simulink model "cocospec_2"  (R2015a)
settings: Solver=ode45  StartTime=0.0  StopTime=10.0  RelTol=1e-3
settings Model: Creator=teme  LastModifiedBy=teme

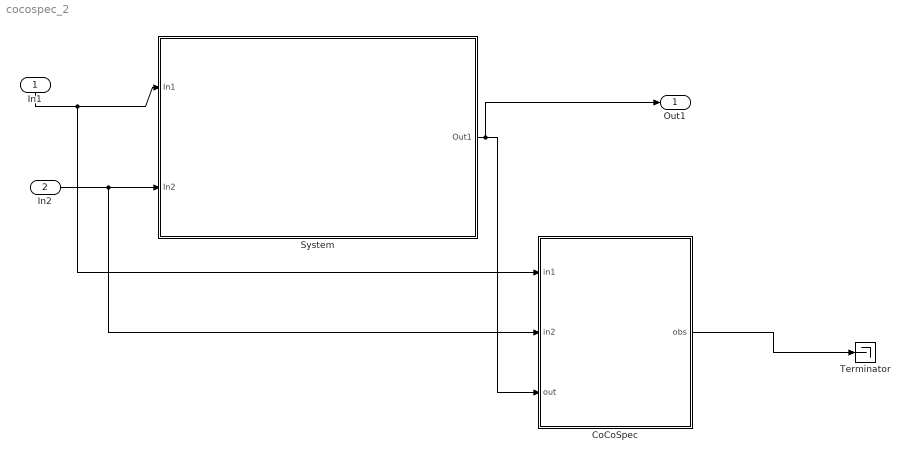
== system cocospec_2 ==
  In1 : Inport  OutDataTypeStr=boolean
  In2 : Inport  Port=2  OutDataTypeStr=double
  CoCoSpec : MATLAB Function  TreatAsAtomicUnit=on
  System : Subsystem
  Terminator : Terminator
  Out1 : Outport
  wires:
  CoCoSpec/1(obs) -> Terminator/1
  In2/1 -> CoCoSpec/2(in2), System/2(In2)
  In1/1 -> CoCoSpec/1(in1), System/1(In1)
  System/1(Out1) -> Out1/1, CoCoSpec/3(out)

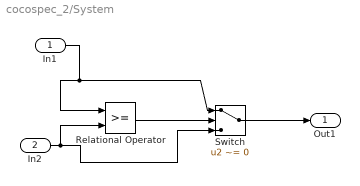
== system cocospec_2/System ==
  In1 : Inport
  In2 : Inport  Port=2
  Relational Operator : RelationalOperator  OutDataTypeStr=boolean
  Switch : Switch  Criteria=u2 ~= 0
  Out1 : Outport
  wires:
  In1/1 -> Relational Operator/1, Switch/1
  In2/1 -> Relational Operator/2, Switch/3
  Relational Operator/1 -> Switch/2
  Switch/1 -> Out1/1

== matlab function cocospec_2/CoCoSpec ==
  data: in1 input; obs output; in2 input; out input
function obs = contract1(in1, in2, out)

%{ 
  assume in1 => 0;
  assume in2 < 10 and in2 => 5; 
%} 

obs = true;

end
